simulink model "cic_test_mdl"  (Simulink 8.1)
settings: Solver=ode45  StartTime=0.0  StopTime=simtime  RelTol=1e-3
values from neighbouring files (symbols this model uses):
  K1 = K1_min    (= 70)    [cic_test.m]    (also in lf_param.m; lf_test.m = 122)
  K2 = K2_min    (= 0.00205994)    [cic_test.m]    (also in lf_param.m = 0.0253754; lf_test.m = 0.1328)
  K3 = K3_min    (= 0.850128)    [cic_test.m]    (also in lf_param.m; lf_test.m = 0.90625)
  mux_sel = 3    [cic_test.m]
  simtime = (length(TS))*ts_in    [cic_test.m]    (also in lf_test.m = (length(lf_in_mat))*ts; param2.m = 1)
  ts_in = 1/625/1e6    (= 1.6e-09)    [cic_test.m]    (also in lf_test.m)
libraries: dspsigops x1
settings Model: MinMaxOverflowLogging=MinMaxAndOverflow  Creator=amr  LastModifiedBy=amr
settings DataIOCC: SignalLoggingSaveFormat=Dataset
settings OptimizationCC: ExpressionDepthLimit=128
settings DebuggingCC: SingleTaskRateTransMsg=error  FcnCallInpInsideContextMsg=EnableAllAsError  LoggingUnavailableSignals=none
settings GRTTargetCC: CombineOutputUpdateFcns=on  GRTInterface=off

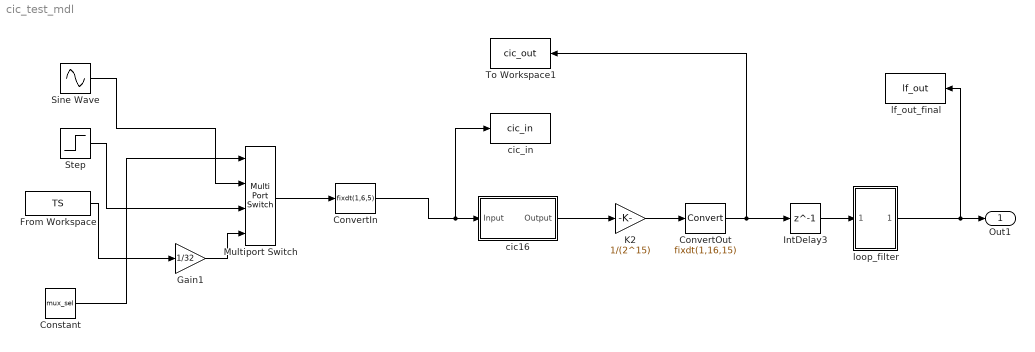
== system cic_test_mdl ==
  Constant : Constant  Value=mux_sel
  ConvertIn : DataTypeConversion  OutDataTypeStr=fixdt(1,6,5)  SampleTime=1/(625e6)  SaturateOnIntegerOverflow=on
  ConvertOut : DataTypeConversion  OutDataTypeStr=fixdt(1,16,15)
  From Workspace : FromWorkspace  VariableName=TS  OutDataTypeStr=double  SampleTime=ts_in  Interpolate=off  OutputAfterFinalValue=Holding final value
  Gain1 : Gain  Gain=1/32  ParamDataTypeStr=double
  IntDelay3 : Delay  DelayLength=1  InitialCondition=0
  K2 : Gain  Gain=1/(2^15)  ParamDataTypeStr=double  OutDataTypeStr=double  SaturateOnIntegerOverflow=on
  Multiport Switch : MultiPortSwitch
  Sine Wave : Sin  Frequency=2*pi*2e6  SampleTime=ts_in
  Step : Step  Time=simtime/2  After=0.5  SampleTime=ts_in
  To Workspace1 : ToWorkspace  VariableName=cic_out  SampleTime=-1
  cic16 : Subsystem  Tag=FilterWizardSubSystem
      settings: ErrorFcn=dspFilterRealizedInBasicElemsAlgLoopErrFcnCallback
  cic_in : ToWorkspace  VariableName=cic_in  SampleTime=-1
  lf_out_final : ToWorkspace  VariableName=lf_out  SampleTime=-1
  loop_filter : Subsystem
  Out1 : Outport
  wires:
  ConvertIn/1 -> cic16/1(Input), cic_in/1
  Step/1 -> Multiport Switch/3
  Sine Wave/1 -> Multiport Switch/2
  From Workspace/1 -> Gain1/1
  Constant/1 -> Multiport Switch/1
  Multiport Switch/1 -> ConvertIn/1
  Gain1/1 -> Multiport Switch/4
  cic16/1(Output) -> K2/1
  ConvertOut/1 -> To Workspace1/1, IntDelay3/1
  K2/1 -> ConvertOut/1
  loop_filter/1(Out1) -> lf_out_final/1, Out1/1
  IntDelay3/1 -> loop_filter/1(In1)

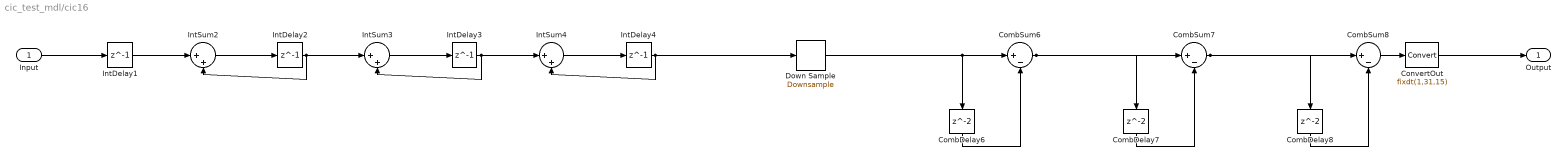
== system cic_test_mdl/cic16 ==
  Input : Inport
  CombDelay6 : Delay  InitialCondition=0
  CombDelay7 : Delay  InitialCondition=0
  CombDelay8 : Delay  InitialCondition=0
  CombSum6 : Sum  Inputs=|+-  AccumDataTypeStr=fixdt(1,21,5)  OutDataTypeStr=fixdt(1,21,5)
  CombSum7 : Sum  Inputs=|+-  AccumDataTypeStr=fixdt(1,21,5)  OutDataTypeStr=fixdt(1,21,5)
  CombSum8 : Sum  Inputs=|+-  AccumDataTypeStr=fixdt(1,21,5)  OutDataTypeStr=fixdt(1,21,5)
  ConvertOut : DataTypeConversion  OutDataTypeStr=fixdt(1,31,15)
  Down Sample : dspsigops/Downsample  N=16  phase=2  RateOptions=Allow multirate processing  smode=Allow multirate  fmode=Maintain input frame size  ic=0
  IntDelay{1..4} (4 alike) : Delay  DelayLength=1  InitialCondition=0
  IntSum2 : Sum  Inputs=|++  AccumDataTypeStr=fixdt(1,21,5)  OutDataTypeStr=fixdt(1,21,5)
  IntSum3 : Sum  Inputs=|++  AccumDataTypeStr=fixdt(1,21,5)  OutDataTypeStr=fixdt(1,21,5)
  IntSum4 : Sum  Inputs=|++  AccumDataTypeStr=fixdt(1,21,5)  OutDataTypeStr=fixdt(1,21,5)
  Output : Outport
  wires:
  Input/1 -> IntDelay1/1
  IntSum2/1 -> IntDelay2/1
  IntDelay2/1 -> IntSum2/2, IntSum3/1
  IntSum3/1 -> IntDelay3/1
  IntDelay3/1 -> IntSum3/2, IntSum4/1
  IntSum4/1 -> IntDelay4/1
  IntDelay4/1 -> IntSum4/2, Down Sample/1
  CombSum6/1 -> CombSum7/1, CombDelay7/1
  CombDelay6/1 -> CombSum6/2
  Down Sample/1 -> CombSum6/1, CombDelay6/1
  CombSum7/1 -> CombSum8/1, CombDelay8/1
  CombDelay7/1 -> CombSum7/2
  CombSum8/1 -> ConvertOut/1
  CombDelay8/1 -> CombSum8/2
  ConvertOut/1 -> Output/1
  IntDelay1/1 -> IntSum2/1

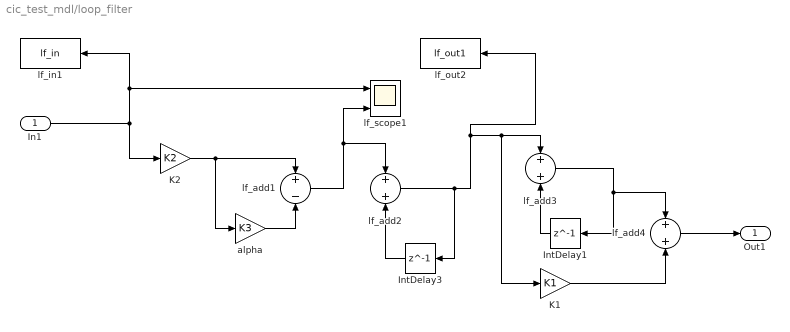
== system cic_test_mdl/loop_filter ==
  In1 : Inport
  IntDelay1 : Delay  DelayLength=1  InitialCondition=0
  IntDelay3 : Delay  DelayLength=1  InitialCondition=0
  K1 : Gain  Gain=K1  ParamDataTypeStr=fixdt(1,9,0)  OutDataTypeStr=fixdt(1,15,10)  SaturateOnIntegerOverflow=on
  K2 : Gain  Gain=K2  ParamDataTypeStr=fixdt(1,5,9)  OutDataTypeStr=fixdt(1,16,20)  SaturateOnIntegerOverflow=on
  alpha : Gain  Gain=K3  ParamDataTypeStr=fixdt(1,10,9)  OutDataTypeStr=fixdt(1,16,20)  SaturateOnIntegerOverflow=on
  lf_add1 : Sum  Inputs=+-  OutDataTypeStr=fixdt(1,16,20)  SaturateOnIntegerOverflow=on
  lf_add2 : Sum  OutDataTypeStr=fixdt(1,16,20)  SaturateOnIntegerOverflow=on
  lf_add3 : Sum  OutDataTypeStr=fixdt(1,15,10)  SaturateOnIntegerOverflow=on
  lf_add4 : Sum  OutDataTypeStr=fixdt(1,15,10)  SaturateOnIntegerOverflow=on
  lf_in1 : ToWorkspace  VariableName=lf_in  SampleTime=-1
  lf_out2 : ToWorkspace  VariableName=lf_out1  SampleTime=-1
  lf_scope1 : Scope  NumInputPorts=2
      settings: TimeRange=1.8e-06  YMin=0~-5  YMax=20~5
  Out1 : Outport
  wires:
  lf_add1/1 -> lf_add2/1, lf_scope1/2
  alpha/1 -> lf_add1/2
  IntDelay3/1 -> lf_add2/2
  K2/1 -> lf_add1/1, alpha/1
  In1/1 -> K2/1, lf_in1/1, lf_scope1/1
  lf_add2/1 -> IntDelay3/1, K1/1, lf_add3/1, lf_out2/1
  IntDelay1/1 -> lf_add3/2
  lf_add3/1 -> lf_add4/1, IntDelay1/1
  K1/1 -> lf_add4/2
  lf_add4/1 -> Out1/1
